simulink model "phase3_scheduler_application4"  (R2026a)
settings: Solver=FixedStepDiscrete  EnableMultiTasking=on
undefined symbols (not defined in the file): phase3_scheduler_application4
libraries: proctasklib x1
settings Model: Creator=The MathWorks, Inc.  LastModifiedBy=rayyu
settings SolverCC: PositivePriorityOrder=on
settings HardwareCC: ProdBitPerLong=64.0  ProdLargestAtomicInteger=LongLong  ProdLargestAtomicFloat=Double  ProdHWDeviceType=ARM Compatible->ARM Cortex-A (64-bit)  HardwareBoardFeatureSet=SoCBlockset
settings RTWCC: SystemTargetFile=ert.tlc  HardwareBoard=Xilinx Zynq UltraScale+ MPSoC ZCU102 Evaluation Kit  TLCOptions="-aInlineSetEventsForThisBaseRateFcn=TLC_FALSE -aSuppressMultiTaskScheduler=TLC_FALSE  -aRateBasedStepFcn=0"  GenerateReport=on  Toolchain=Linaro AArch64 Linux v6.3.1  IncludeHyperlinkInReport=on  LaunchReport=on  GenerateTraceInfo=on  GenerateTraceReport=on  GenerateTraceReportSl=on  GenerateTraceReportSf=on  GenerateTraceReportEml=on  Description=Embedded Coder
settings ERTTargetCC: ExtModeTransport=2.0  DynamicArrayContainerType=coder::array

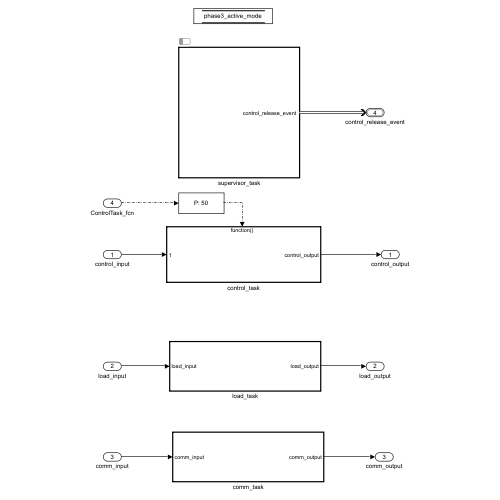
[thumbnail: Simulink's stored preview of the top-level diagram]
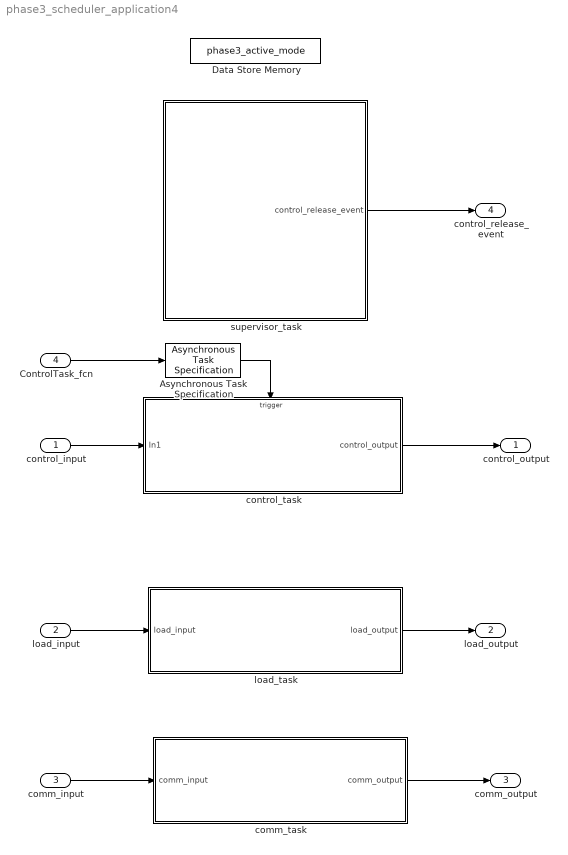
== system phase3_scheduler_application4 ==
  control_input : Inport
  load_input : Inport  Port=2  SampleTime=0.05  Interpolate=off
  comm_input : Inport  Port=3  SampleTime=0.005  Interpolate=off
  ControlTask_fcn : Inport  Port=4  OutputFunctionCall=on
  Asynchronous Task Specification : AsynchronousTaskSpecification  TaskPriority=50
  Data Store Memory : DataStoreMemory  DataStoreName=phase3_active_mode  WriteAfterWriteMsg=warning  InitialValue=3  ShowAdditionalParam=off  OutDataTypeStr=uint8
  comm_task : Subsystem  TreatAsAtomicUnit=on
  control_task : Subsystem  TreatAsAtomicUnit=on
  load_task : Subsystem  TreatAsAtomicUnit=on
  supervisor_task : Subsystem  TreatAsAtomicUnit=on  ScheduleAs=Periodic partition  PartitionName=SupervisorTask  SystemSampleTime=0.01
  control_output : Outport  VectorParamsAs1DForOutWhenUnconnected=off
  load_output : Outport  Port=2  VectorParamsAs1DForOutWhenUnconnected=off
  comm_output : Outport  Port=3
  control_release_event : Outport  InputPortMessageModes=m  Port=4  OutDataTypeStr=Bus: rteEvent  BusOutputAsStruct=on
  wires:
  control_task/1(control_output) -> control_output/1
  control_input/1 -> control_task/1(In1)
  load_input/1 -> load_task/1(load_input)
  load_task/1(load_output) -> load_output/1
  comm_input/1 -> comm_task/1(comm_input)
  comm_task/1(comm_output) -> comm_output/1
  supervisor_task/1("control_release_event ") -> control_release_event/1
  ControlTask_fcn/1 -> Asynchronous Task Specification/1
  Asynchronous Task Specification/1 -> control_task/Trigger

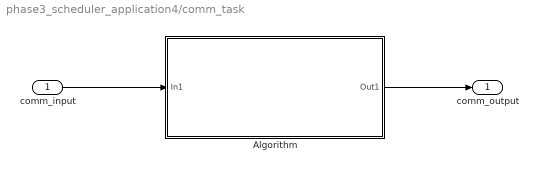
== system phase3_scheduler_application4/comm_task ==
  comm_input : Inport
  Algorithm : Subsystem
  comm_output : Outport  VectorParamsAs1DForOutWhenUnconnected=off
  wires:
  comm_input/1 -> Algorithm/1(In1)
  Algorithm/1(Out1) -> comm_output/1

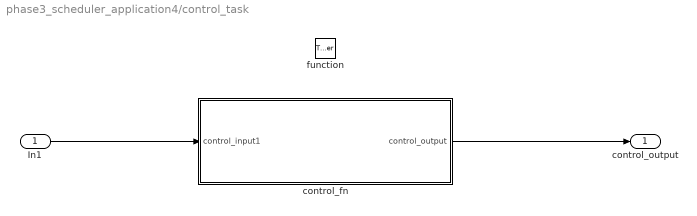
== system phase3_scheduler_application4/control_task ==
  In1 : Inport
  function : TriggerPort  TriggerType=function-call  VariantControl=(inherit)
  control_fn : Subsystem  TreatAsAtomicUnit=on
  control_output : Outport
  wires:
  In1/1 -> control_fn/1(control_input1)
  control_fn/1(control_output) -> control_output/1

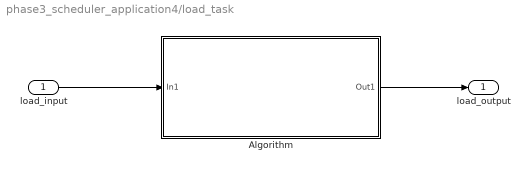
== system phase3_scheduler_application4/load_task ==
  load_input : Inport
  Algorithm : Subsystem
  load_output : Outport  VectorParamsAs1DForOutWhenUnconnected=off
  wires:
  Algorithm/1(Out1) -> load_output/1
  load_input/1 -> Algorithm/1(In1)

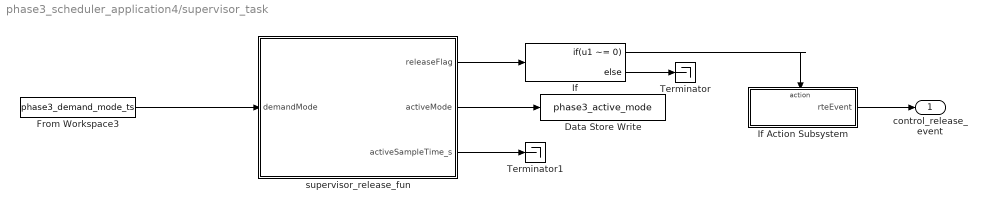
== system phase3_scheduler_application4/supervisor_task ==
  Data Store Write : DataStoreWrite  DataStoreName=phase3_active_mode  IndexOptions=Index vector (dialog)  Indices=1  OutputSizes=1
  From Workspace3 : FromWorkspace  VariableName=phase3_demand_mode_ts  SampleTime=-1  Interpolate=off  OutputAfterFinalValue=Holding final value
  If : If  IfExpression=u1 ~= 0
  If Action Subsystem : Subsystem  TreatAsAtomicUnit=on
  Terminator : Terminator
  Terminator1 : Terminator
  supervisor_release_fun : MATLAB Function  TreatAsAtomicUnit=on
  "control_release_event " : Outport  OutDataTypeStr=Bus: rteEvent
  wires:
  From Workspace3/1 -> supervisor_release_fun/1(demandMode)
  supervisor_release_fun/1(releaseFlag) -> If/1
  supervisor_release_fun/2(activeMode) -> Data Store Write/1
  supervisor_release_fun/3(activeSampleTime_s) -> Terminator1/1
  If/1 -> If Action Subsystem/Action
  If/2 -> Terminator/1
  If Action Subsystem/1(rteEvent) -> "control_release_event "/1

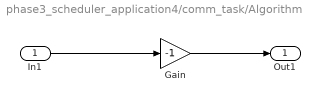
== system phase3_scheduler_application4/comm_task/Algorithm ==
  In1 : Inport
  Gain : Gain  Gain=-1
  Out1 : Outport  VectorParamsAs1DForOutWhenUnconnected=off
  wires:
  Gain/1 -> Out1/1
  In1/1 -> Gain/1

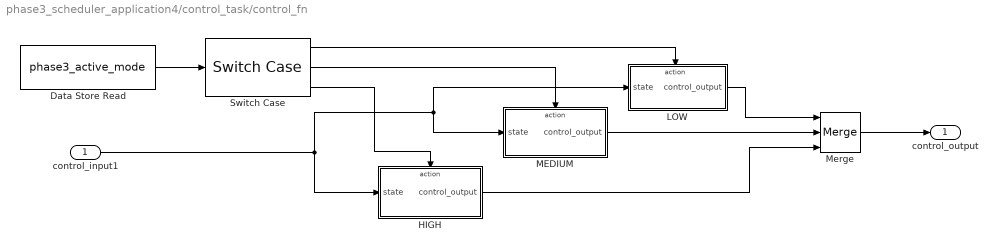
== system phase3_scheduler_application4/control_task/control_fn ==
  control_input1 : Inport
  Data Store Read : DataStoreRead  DataStoreName=phase3_active_mode  IndexOptions=Index vector (dialog)  Indices=1  OutputSizes=1
  HIGH : Subsystem  TreatAsAtomicUnit=on
  LOW : Subsystem  TreatAsAtomicUnit=on
  MEDIUM : Subsystem  TreatAsAtomicUnit=on
  Merge : Merge  Inputs=3
  Switch Case : SwitchCase  CaseConditions={1, 2, 3}  ShowDefaultCase=off
  control_output : Outport
  wires:
  control_input1/1 -> LOW/1(state), MEDIUM/1(state), HIGH/1(state)
  Data Store Read/1 -> Switch Case/1
  Switch Case/1 -> LOW/Action
  Switch Case/2 -> MEDIUM/Action
  Switch Case/3 -> HIGH/Action
  LOW/1(control_output) -> Merge/1
  MEDIUM/1(control_output) -> Merge/2
  HIGH/1(control_output) -> Merge/3
  Merge/1 -> control_output/1

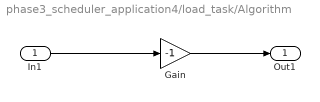
== system phase3_scheduler_application4/load_task/Algorithm ==
  In1 : Inport
  Gain : Gain  Gain=-1
  Out1 : Outport  VectorParamsAs1DForOutWhenUnconnected=off
  wires:
  In1/1 -> Gain/1
  Gain/1 -> Out1/1

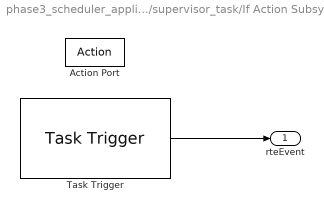
== system phase3_scheduler_application4/supervisor_task/If Action Subsystem ==
  Action Port : ActionPort  ActionPortLabel=if(u1 ~= 0)
  Task Trigger : proctasklib/Task Trigger  BlockSID=phase3_scheduler_application4:90
  rteEvent : Outport
  wires:
  Task Trigger/1 -> rteEvent/1

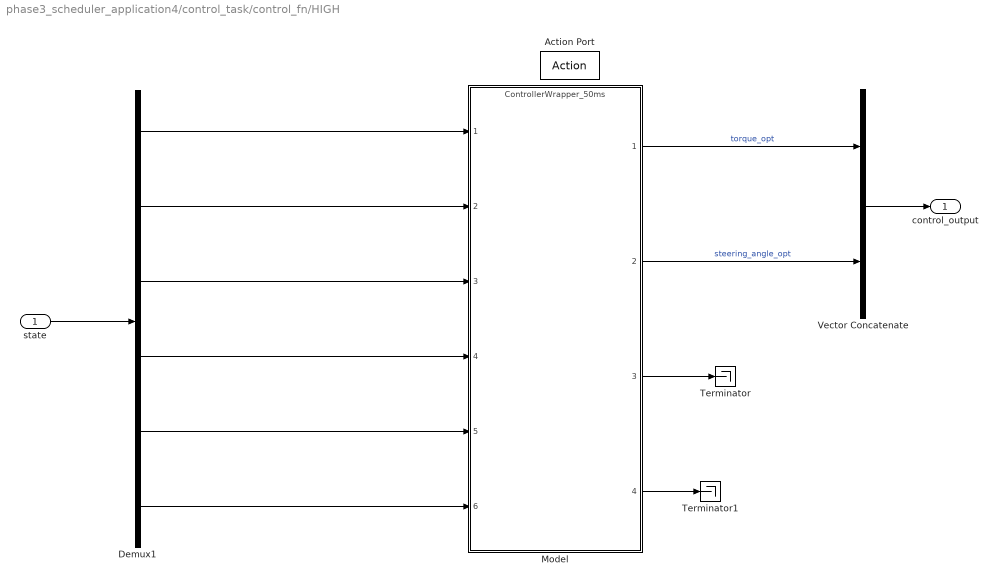
== system phase3_scheduler_application4/control_task/control_fn/HIGH ==
  state : Inport
  Action Port : ActionPort  ActionPortLabel=case [ 3 ]:
  Demux1 : Demux  Outputs=6
  Model : ModelReference  ModelNameDialog=ControllerWrapper_50ms.slx  SimulationMode=Normal  ModelReferenceVersion=1.48
  Terminator : Terminator
  Terminator1 : Terminator
  Vector Concatenate : Concatenate
  control_output : Outport
  wires:
  Demux1/3 -> Model/3
  Demux1/2 -> Model/2
  Demux1/6 -> Model/6
  Demux1/1 -> Model/1
  state/1 -> Demux1/1
  Demux1/5 -> Model/5
  Demux1/4 -> Model/4
  Model/2 -> Vector Concatenate/2  "steering_angle_opt"
  Model/1 -> Vector Concatenate/1  "torque_opt"
  Vector Concatenate/1 -> control_output/1
  Model/3 -> Terminator/1
  Model/4 -> Terminator1/1

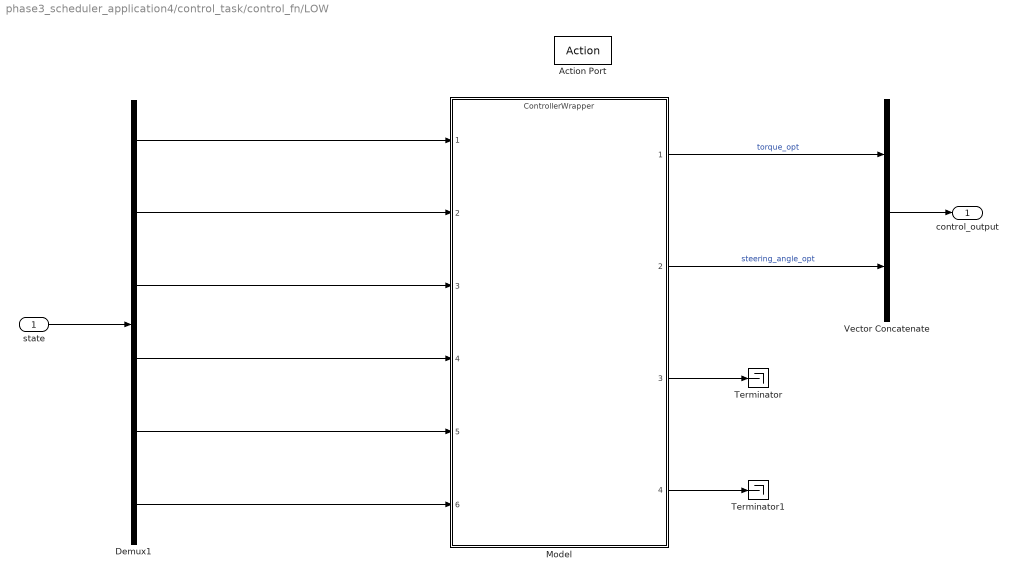
== system phase3_scheduler_application4/control_task/control_fn/LOW ==
  state : Inport
  Action Port : ActionPort  ActionPortLabel=case [ 1 ]:
  Demux1 : Demux  Outputs=6
  Model : ModelReference  ModelNameDialog=ControllerWrapper.slx  SimulationMode=Normal  ModelReferenceVersion=1.48
  Terminator : Terminator
  Terminator1 : Terminator
  Vector Concatenate : Concatenate
  control_output : Outport
  wires:
  Demux1/3 -> Model/3
  Demux1/2 -> Model/2
  Demux1/6 -> Model/6
  Demux1/1 -> Model/1
  state/1 -> Demux1/1
  Demux1/5 -> Model/5
  Demux1/4 -> Model/4
  Model/2 -> Vector Concatenate/2  "steering_angle_opt"
  Model/1 -> Vector Concatenate/1  "torque_opt"
  Vector Concatenate/1 -> control_output/1
  Model/3 -> Terminator/1
  Model/4 -> Terminator1/1

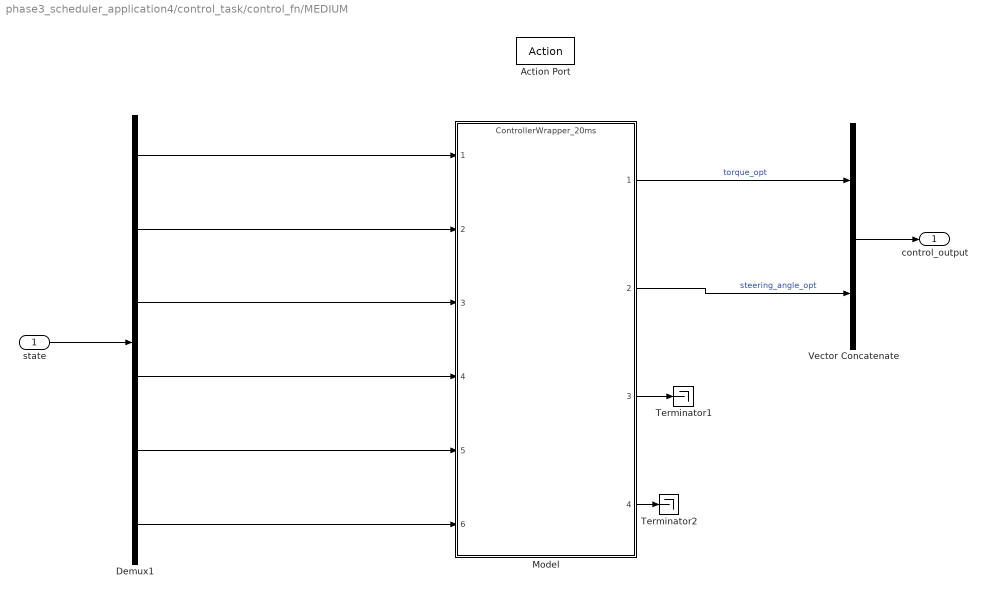
== system phase3_scheduler_application4/control_task/control_fn/MEDIUM ==
  state : Inport
  Action Port : ActionPort  ActionPortLabel=case [ 2 ]:
  Demux1 : Demux  Outputs=6
  Model : ModelReference  ModelNameDialog=ControllerWrapper_20ms.slx  SimulationMode=Normal  ModelReferenceVersion=1.48
  Terminator1 : Terminator
  Terminator2 : Terminator
  Vector Concatenate : Concatenate
  control_output : Outport
  wires:
  Demux1/3 -> Model/3
  Demux1/2 -> Model/2
  Demux1/6 -> Model/6
  Demux1/1 -> Model/1
  state/1 -> Demux1/1
  Demux1/5 -> Model/5
  Demux1/4 -> Model/4
  Model/3 -> Terminator1/1
  Model/4 -> Terminator2/1
  Model/2 -> Vector Concatenate/2  "steering_angle_opt"
  Model/1 -> Vector Concatenate/1  "torque_opt"
  Vector Concatenate/1 -> control_output/1

== matlab function phase3_scheduler_application4/supervisor_task/supervisor_release_fun ==
  data: demandMode input; releaseFlag output; activeMode output; activeSampleTime_s output
function [ ...
    releaseFlag, ...
    activeMode, ...
    activeSampleTime_s] = ...
    supervisorReleaseLogic(demandMode)

persistent ticksRemaining
persistent latchedMode

if isempty(ticksRemaining)
    ticksRemaining = uint8(0);
    latchedMode = uint8(3);
end

% LOW = 50 ms, MEDIUM = 20 ms, HIGH = 10 ms.
periodTicks = uint8([5; 2; 1]); % number of ticks before it triggers the controller

requestedMode = uint8( ...
    min(max(double(demandMode), 1), 3));

% Escalate immediately when demand increases.
if requestedMode > latchedMode
    ticksRemaining = uint8(0);
end

releaseFlag = ticksRemaining == 0; % release controller

if releaseFlag

    % Mode changes occur only at a controller release.
    latchedMode = requestedMode;

    ticksRemaining = ...
        periodTicks(double(latchedMode)) - uint8(1);

else
    ticksRemaining = ticksRemaining - uint8(1);
end

activeMode = latchedMode;

activeSampleTime_s = ...
    0.010 * double(periodTicks(double(activeMode)));

end
